simulink model "threephasePWMRectifier_open"  (R2017b)
settings: Solver=ode23  StartTime=0.0  StopTime=0.3  RelTol=1e-3  EnableMultiTasking=on
undefined symbols (not defined in the file): DiscIntNeverNeededParam, Vdc_Ref
libraries: powerlib x15, powerlib_extras x7, simulink x2
settings Model: Creator=ztm  LastModifiedBy=陈鹏旺
settings DataIOCC: LimitDataPoints=on  SaveFormat=Array  SignalLoggingSaveFormat=ModelDataLogs
settings OptimizationCC: ExpressionDepthLimit=2147483647  LifeSpan=inf
settings DebuggingCC: UnderspecifiedInitializationDetection=Classic  MergeDetectMultiDrivingBlocksExec=none  SolverPrmCheckMsg=warning  FcnCallInpInsideContextMsg=warning  StateNameClashWarn=warning  SFUnexpectedBacktrackingDiag=warning  SFNoUnconditionalDefaultTransitionDiag=warning  SFExecutionAtInitializationDiag=none
settings HardwareCC: ProdBitPerPointer=32  ProdBitPerSizeT=32  ProdBitPerPtrDiffT=32  ProdLargestAtomicFloat=None  ProdIntDivRoundTo=Undefined  ProdEndianess=Unspecified  ProdWordSize=32  ProdHWDeviceType=32-bit Generic
settings ModelReferenceCC: PropagateSignalLabelsOutOfModel=off
settings CodeAppCC: StateflowObjectComments=on
settings GRTTargetCC: TargetLangStandard=C89/C90 (ANSI)  GeneratePreprocessorConditionals=Disable all  CombineOutputUpdateFcns=off  GRTInterface=on
settings ConfigComp: CovMetricSettings=dw  CovHtmlReporting=on  CovSaveCumulativeToWorkspaceVar=on  CovSaveSingleToWorkspaceVar=on  CovExternalEMLEnable=off
settings SimscapeCC: SimscapeNormalizeSystem=off

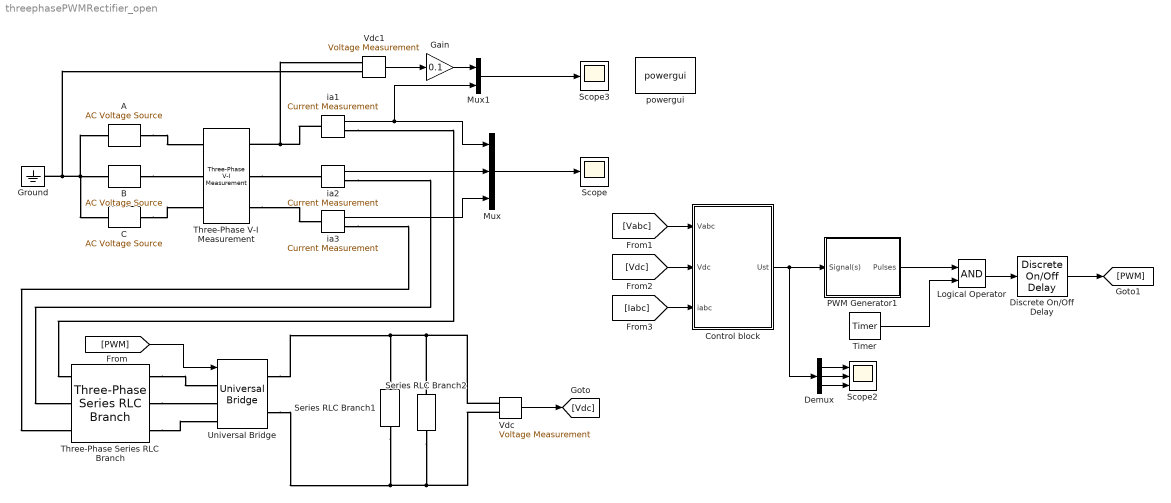
== system threephasePWMRectifier_open ==
  A : powerlib/Electrical Sources/AC Voltage Source  Amplitude=130*sqrt(2)/sqrt(3)  Phase=0  Frequency=50  SampleTime=0  Measurements=Voltage  BusType=swing  Pref=10e3  Qref=0  Qmin=-inf  Qmax=+inf
  B : powerlib/Electrical Sources/AC Voltage Source  Amplitude=130*sqrt(2)/sqrt(3)  Phase=-120  Frequency=50  SampleTime=0  Measurements=Voltage  BusType=swing  Pref=10e3  Qref=0  Qmin=-inf  Qmax=+inf
  C : powerlib/Electrical Sources/AC Voltage Source  Amplitude=130*sqrt(2)/sqrt(3)  Phase=120  Frequency=50  SampleTime=0  Measurements=Voltage  BusType=swing  Pref=10e3  Qref=0  Qmin=-inf  Qmax=+inf
  Control block : Subsystem  mask(DC Regulator){Vdc_Ref=280, =Vdc_Ref, Par_VdcReg=[0.8 0.008], Par_IReg=[20 0.0001 0], Par_Nom=[130 605], Ts=1/9000/2, h_I=[10.5 0]}
      mask prompts: Vdc_Ref "DC Voltage setpoint (Volts)";  "DC Voltage setpoint (Volts)"; Par_VdcReg "Vdc Regulator Gains: [ Kp  Ki]"; Par_IReg "Current Regulators Gain: [ Kp Ki Kr ]"; Par_Nom "Nominal Voltage and power: [ Vnom (volts rms L-L)  Pnom (VA) ]"; Ts "Time Step (s)"; h_I "[kph kih]"
      mask init:
      | Vnom=Par_Nom(1);
      | Pnom=Par_Nom(2);
      | Kp_I=Par_IReg(1);
      | Ki_I=Par_IReg(2);
      | Kr=Par_IReg(3);
      | Kp_Vdc=Par_VdcReg(1);
      | Ki_Vdc=Par_VdcReg(2);
      | Kph_I=h_I(1);
      | Kih_I=h_I(2);
  Demux : Demux  Outputs=3
  Discrete On/Off Delay : powerlib_extras/Discrete  Control Blocks/Discrete On//Off Delay  type_delay=On delay  delay=5e-6  ic=0  Ts=3.9e-7
  Gain : Gain  Gain=0.1
  Ground : powerlib/Elements/Ground  LConnTagsString=a
  Logical Operator : Logic  AllPortsSameDT=off  OutDataTypeStr=boolean
  Mux : Mux  Inputs=3
  Mux1 : Mux  Inputs=2
  PWM Generator1 : Subsystem  AncestorBlock="powerlib_extras/Control  Blocks/PWM Generator"  DialogController=POWERSYS.PowerSysDialog  mask(PWM Generator){GeneratorMode=3-arm  bridge (6 pulses), Fc=9000, Internal=off, mIndex=0.2, Freq=50, Phase=60}
      mask prompts: GeneratorMode "Generator Mode"; Fc "Carrier frequency (Hz):"; Internal "Internal generation of modulating signal(s)"; mIndex "Modulation index  (0<m<1) :"; Freq "Frequency of output voltage (Hz)"; Phase "Phase of output voltage (degrees)"
      mask help:
      | This block generates pulses for carrier-based PWM (Pulse Width Modulation), self-commutated IGBTs,GTOs or FETs bridges.
      |
      | Depending on the number of bridge arms selected in the "Generator Mode" parameter, the block can be used either for single-phase or three-phase PWM control.
      mask init:
      | powericon('psbcallbacks',gcb,'PWM Generator');
      | if Freq==0
      |     Phase=90;
      | end
      | switch GeneratorMode
      | case 1,
      |     Internal_Phase=0;
      |    Signal_PortWidth=1;
      |    Select1_Elements=[1 2];
      |    Select1_PortWidth=2;
      |    Select3_Elements=[1 2];
      |    Select3_PortWidth=4;
      | case 2,
      |     Internal_Phase=0;
      |     Signal_PortWidth=1;
      |     Select1_Elements=[1 2];
      |     Select1_PortWidth=2;
      |     Select3_Elements=[1 2 3 4];
      |     Select3_PortWidth=4;
      | case 3,
      |     Internal_Phase=[0 -2*pi/3 2*pi/3];
      |     Signal_PortWidth=3;
      |     Select1_Elements=[1 4 2 5 3 6];
      |     Select1_PortWidth=6;
      |    Select3_Elements=[1 2 3 4 5 6];
      |    Select3_PortWidth=12;
      | case 4,
      |     Internal_Phase=[0 -2*pi/3 2*pi/3];
      |     Signal_PortWidth=3;
      |     Select1_Elements=[1 4 2 5 3 6];
      |     Select1_PortWidth=6;
      |    Select3_Elements=[1 2 3 4 5 6 7 8 9 10 11 12];
      |    Select3_PortWidth=12;
      | end
      | power_initmask();
      mask Help: web(psbhelp)
      mask TypeOptions GeneratorMode: 1-arm  bridge (2 pulses) | 2-arm  bridge (4 pulses) | 3-arm  bridge (6 pulses) | Double 3-arm  bridges (12 pulses)
  Scope : Scope
  Scope2 : Scope  NumInputPorts=3
  Scope3 : Scope
  Series RLC Branch1 : powerlib/Elements/Series RLC Branch  LConnTagsString=__new0  RConnTagsString=__new0  BranchType=C  Resistance=20  Inductance=1e-5  SetiL0=off  InitialCurrent=0  Capacitance=2e-3  Setx0=on  InitialVoltage=252  Measurements=None
  Series RLC Branch2 : powerlib/Elements/Series RLC Branch  LConnTagsString=__new0  RConnTagsString=__new0  BranchType=R  Resistance=60  Inductance=1e-5  SetiL0=off  InitialCurrent=0  Capacitance=1e-6  Setx0=off  InitialVoltage=0  Measurements=None
  Three-Phase Series RLC Branch : powerlib/Elements/Three-Phase Series RLC Branch  LConnTagsString=A|B|C  RConnTagsString=A|B|C  BranchType=RL  Resistance=1e-4  Inductance=2e-3  Capacitance=1e-6  Measurements=None
  Three-Phase V-I Measurement : powerlib/Measurements/Three-Phase V-I Measurement  VoltageMeasurement=phase-to-ground  SetLabelV=on  LabelV=Vabc  Vpu=off  VpuLL=off  CurrentMeasurement=yes  SetLabelI=on  LabelI=Iabc  Ipu=off  Pbase=100e6  Vbase=500e3  OutputType=Complex  PhasorSimulation=off  PSBequivalent=0
  Timer : powerlib_extras/Control  Blocks/Timer  t=[0 0.001]  e=[0 1]
  Universal Bridge : powerlib/Power Electronics/Universal Bridge  Arms=3  SnubberResistance=1e6  SnubberCapacitance=inf  Device=MOSFET / Diodes  Ron=11e-3  Lon=0  ForwardVoltages="[  0  0  ]"  ForwardVoltage=0  GTOparameters=[ 10e-6 , 20e-6 ]  IGBTparameters=[ 1e-6 , 2e-6 ]  Measurements=None  Measurements_2=None  converterType=Rectifier
  Vdc : powerlib/Measurements/Voltage Measurement  PhasorSimulation=off  OutputType=Complex  PSBequivalent=0
  Vdc1 : powerlib/Measurements/Voltage Measurement  PhasorSimulation=off  OutputType=Complex  PSBequivalent=0
  ia1 : powerlib/Measurements/Current Measurement  PhasorSimulation=off  OutputType=Complex  PSBequivalent=0
  ia2 : powerlib/Measurements/Current Measurement  PhasorSimulation=off  OutputType=Complex  PSBequivalent=0
  ia3 : powerlib/Measurements/Current Measurement  PhasorSimulation=off  OutputType=Complex  PSBequivalent=0
  powergui : powerlib/powergui  Priority=1  SimulationMode=Discrete  SampleTime=3.9e-7  frequency=60  Iterations=50  frequencyindice=50  Pbase=100e6  ErrMax=1e-4  UnitsV=kV  UnitsW=MW  buscounter=0  FunctionMessages=off  echomessages=off  EnableUseOfTLC=off  CurrentSourceSwitches=off  DisableSnubberDevices=off  DisableRonSwitches=off  DisableVfSwitches=off  DisplayEquations=off  SolverType=Tustin/Backward Euler (TBE)  Interpol=off  ExternalGateDelay=off  methode=off  Ts=0  x0status=blocks  SPID=off  SwTol=0  HookPort=off  RestoreLinks=warning  ResistiveCurrentMeasurement=off  Frange=[0:2:500]  Ylog=off  Xlog=on  ShowGrid=off  save=off  variable=ZData  structure=ScopeData  ZoomFFT=off  StartTime=0.15  cycles=3  DisplayStyle=2  fundamental=50  FreqAxis=off  MaxFrequency=9000  frequencyindicesteady=1  RmsSteady=1  display=off
  wires:
  Vdc/1 -> [Vdc]
  Mux/1 -> Scope/1
  [Vabc] -> Control block/1(Vabc)
  [Vdc] -> Control block/2(Vdc)
  [Iabc] -> Control block/3(iabc)
  Control block/1(Ust) -> Demux/1, PWM Generator1/1(Signal(s))
  Demux/1 -> Scope2/1
  Demux/2 -> Scope2/2
  Demux/3 -> Scope2/3
  Timer/1 -> Logical Operator/2
  Logical Operator/1 -> Discrete On/Off Delay/1
  Vdc1/1 -> Gain/1
  Gain/1 -> Mux1/1
  Mux1/1 -> Scope3/1
  ia1/1 -> Mux/1, Mux1/2
  ia3/1 -> Mux/3
  ia2/1 -> Mux/2
  Discrete On/Off Delay/1 -> [PWM]
  PWM Generator1/1(Pulses) -> Logical Operator/1
  [PWM] -> Universal Bridge/1
  connections:
  C/LConn1 -- B/LConn1 -- A/LConn1 -- Ground/LConn1 -- Vdc1/LConn2
  B/RConn1 -- Three-Phase V-I Measurement/LConn2
  A/RConn1 -- Three-Phase V-I Measurement/LConn1
  C/RConn1 -- Three-Phase V-I Measurement/LConn3
  ia1/LConn1 -- Three-Phase V-I Measurement/RConn1 -- Vdc1/LConn1
  Three-Phase V-I Measurement/RConn3 -- ia3/LConn1
  Three-Phase V-I Measurement/RConn2 -- ia2/LConn1
  Vdc/LConn2 -- Series RLC Branch2/RConn1 -- Universal Bridge/RConn2 -- Series RLC Branch1/RConn1
  Three-Phase Series RLC Branch/RConn1 -- Universal Bridge/LConn1
  Three-Phase Series RLC Branch/RConn2 -- Universal Bridge/LConn2
  Three-Phase Series RLC Branch/RConn3 -- Universal Bridge/LConn3
  ia1/RConn1 -- Three-Phase Series RLC Branch/LConn1
  ia2/RConn1 -- Three-Phase Series RLC Branch/LConn2
  ia3/RConn1 -- Three-Phase Series RLC Branch/LConn3
  Vdc/LConn1 -- Series RLC Branch2/LConn1 -- Series RLC Branch1/LConn1 -- Universal Bridge/RConn1

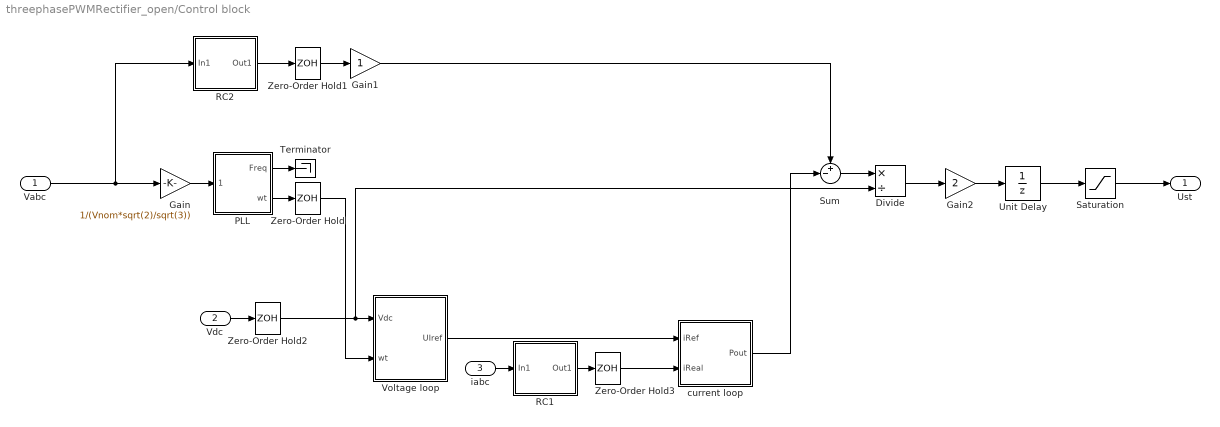
== system threephasePWMRectifier_open/Control block ==
  Vabc : Inport
  Vdc : Inport  Port=2
  iabc : Inport  Port=3
  Divide : Product  Inputs=*/
  Gain : Gain  Gain=1/(Vnom*sqrt(2)/sqrt(3))
  Gain1 : Gain
  Gain2 : Gain  Gain=2
  PLL : Subsystem  AncestorBlock=|  mask(Discrete 3-phase PLL){Fmin=-48, Par_Init=[0 50], ParK=[100 140], Ts=Ts, AGC=off}
      | powerlib_extras/Discrete 
      | Control Blocks/Discrete
      | 3-phase PLL
      mask prompts: Fmin "Minimum frequency (Hz):"; Par_Init "Initial inputs:[ Phase(degrees)   Frequency(Hz) ]"; ParK "Regulator gains [ Kp  Ki  Kd ]"; Ts "Sample time:"; AGC "Enable Automatic Gain Control"
      mask help:
      | This Phase Locked Loop (PLL) system can be used  to synchronize on a set of variable frequency, three-phase sinusoidal signals. If the Automatic Gain Control is enabled, the input (phase error) of the PLL regulator is scaled according to the input signals magnitude.
      |
      | For optimal performance, the following settings are recommended:
      |   [ Kp Ki  Kd ] = [ 180  3200  1 ]
      |   "Enable Automatic Gain Control" checked
      |
      | Input 1: Vector containing the normalized three-phase signals [Va Vb Vc]
      | Output 1:  Measured frequency (Hz) = w/(2pi)
      | Output 2:  Ramp w.t varying between  0 and 2*pi,
      |      synchronized on zero crossings of the fundamental (positive-sequence) of phase A.
      | Output 3: Vector [sin(wt) cos(wt)]
      mask init:
      | Kp=ParK(1);
      | Ki=ParK(2);
      | if length(ParK)==2
      |     Kd=0;
      | else
      |     Kd=ParK(3);
      | end    
      | Phase_Init=Par_Init(1);
      | Finit=Par_Init(2);
      | power_initmask();
      settings: OpenFcn=power_openblockproxy();
  RC1 : Subsystem
  RC2 : Subsystem
  Saturation : Saturate  UpperLimit=0.98  LowerLimit=-0.98
  Sum : Sum  Inputs=+-|
  Terminator : Terminator
  Unit Delay : UnitDelay  SampleTime=Ts/2
  Voltage loop : Subsystem
  Zero-Order Hold{,1..3} (4 alike) : ZeroOrderHold  SampleTime=Ts
  current loop : Subsystem
  Ust : Outport
  wires:
  Gain/1 -> PLL/1(Vabc(pu))
  PLL/1(Freq) -> Terminator/1
  PLL/2(wt) -> Zero-Order Hold/1
  RC2/1(Out1) -> Zero-Order Hold1/1
  Zero-Order Hold1/1 -> Gain1/1
  Vdc/1 -> Zero-Order Hold2/1
  Zero-Order Hold/1 -> Voltage loop/2(wt)
  Zero-Order Hold2/1 -> Voltage loop/1(Vdc), Divide/2
  iabc/1 -> RC1/1(In1)
  RC1/1(Out1) -> Zero-Order Hold3/1
  Gain1/1 -> Sum/1
  Sum/1 -> Divide/1
  Divide/1 -> Gain2/1
  Gain2/1 -> Unit Delay/1
  Saturation/1 -> Ust/1
  Vabc/1 -> Gain/1, RC2/1(In1)
  Zero-Order Hold3/1 -> current loop/2(iReal)
  Unit Delay/1 -> Saturation/1
  current loop/1(Pout) -> Sum/2
  Voltage loop/1(UIref) -> current loop/1(iRef)

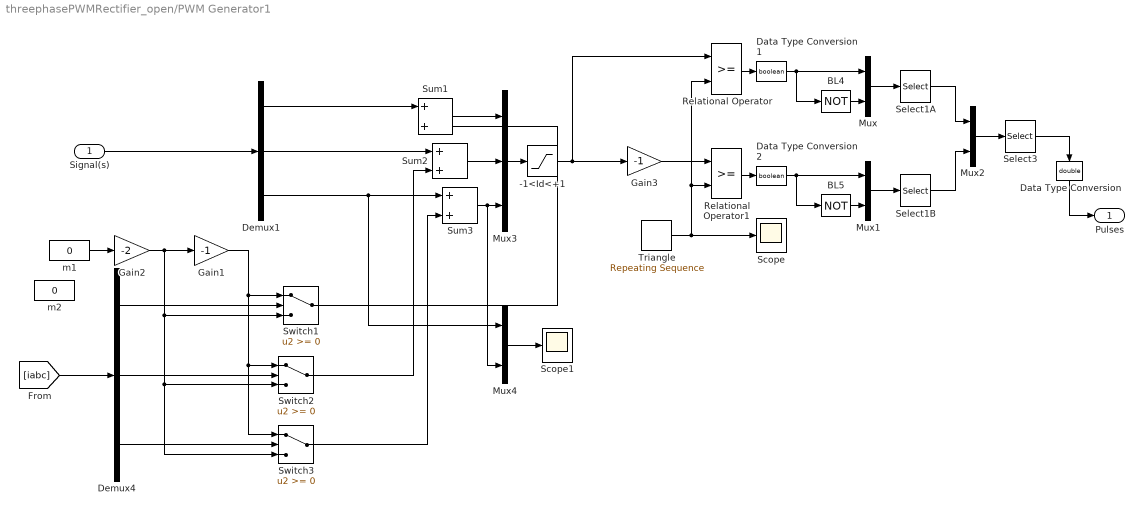
== system threephasePWMRectifier_open/PWM Generator1 ==
  Signal(s) : Inport
  -1<Id<+1 : Saturate  UpperLimit=0.94  LowerLimit=-0.94
  BL4 : Logic  Operator=NOT  Inputs=1
  BL5 : Logic  Operator=NOT  Inputs=1
  Data Type Conversion : DataTypeConversion  OutDataTypeStr=double  SaturateOnIntegerOverflow=on  RndMeth=Zero
  Data Type Conversion1 : DataTypeConversion  OutDataTypeStr=boolean  SaturateOnIntegerOverflow=on  RndMeth=Zero
  Data Type Conversion2 : DataTypeConversion  OutDataTypeStr=boolean  SaturateOnIntegerOverflow=on  RndMeth=Zero
  Demux1 : Demux  Outputs=3
  Demux4 : Demux  Outputs=3
  Gain1 : Gain  Gain=-1  SaturateOnIntegerOverflow=on  OutDataTypeStr=Inherit: Same as input  ParamDataTypeStr=Inherit: Same as input
  Gain2 : Gain  Gain=-2  SaturateOnIntegerOverflow=on  OutDataTypeStr=Inherit: Same as input  ParamDataTypeStr=Inherit: Same as input
  Gain3 : Gain  Gain=-1  SaturateOnIntegerOverflow=on  OutDataTypeStr=Inherit: Same as input  ParamDataTypeStr=Inherit: Same as input
  Mux{,1..2,4} (4 alike) : Mux  Inputs=2
  Mux3 : Mux  Inputs=3
  Relational Operator : RelationalOperator  RndMeth=Nearest  InputSameDT=on
  Relational Operator1 : RelationalOperator  RndMeth=Nearest  InputSameDT=on
  Scope : Scope
  Scope1 : Scope
  Select1A : Selector  InputPortWidth=Select1_PortWidth  IndexOptions=Index vector (dialog)  Indices=Select1_Elements  OutputSizes=1
  Select1B : Selector  InputPortWidth=Select1_PortWidth  IndexOptions=Index vector (dialog)  Indices=Select1_Elements  OutputSizes=1
  Select3 : Selector  InputPortWidth=Select3_PortWidth  IndexOptions=Index vector (dialog)  Indices=Select3_Elements  OutputSizes=1
  Sum1 : Sum  SaturateOnIntegerOverflow=on  InputSameDT=on  OutDataTypeStr=Inherit: Same as first input
  Sum2 : Sum  SaturateOnIntegerOverflow=on  InputSameDT=on  OutDataTypeStr=Inherit: Same as first input
  Sum3 : Sum  SaturateOnIntegerOverflow=on  InputSameDT=on  OutDataTypeStr=Inherit: Same as first input
  Switch1 : Switch  InputSameDT=on
  Switch2 : Switch  InputSameDT=on
  Switch3 : Switch  InputSameDT=on
  Triangle : simulink/Sources/Repeating Sequence  rep_seq_t=[0 1/Fc/4 3/Fc/4 1/Fc]  rep_seq_y=[0 -1 1 0]
  m1 : Constant  Value=0
  m2 : Constant  Value=0
  Pulses : Outport
  wires:
  Data Type Conversion2/1 -> Mux1/1, BL5/1
  Relational Operator1/1 -> Data Type Conversion2/1
  Data Type Conversion1/1 -> Mux/1, BL4/1
  Relational Operator/1 -> Data Type Conversion1/1
  Data Type Conversion/1 -> Pulses/1
  Select3/1 -> Data Type Conversion/1
  Gain3/1 -> Relational Operator1/1
  BL4/1 -> Mux/2
  BL5/1 -> Mux1/2
  Mux/1 -> Select1A/1
  Mux1/1 -> Select1B/1
  Select1A/1 -> Mux2/1
  Select1B/1 -> Mux2/2
  Mux2/1 -> Select3/1
  Triangle/1 -> Relational Operator1/2, Relational Operator/2, Scope/1
  [iabc] -> Demux4/1
  Demux4/1 -> Switch1/2
  Gain1/1 -> Switch1/1, Switch2/1, Switch3/1
  Demux4/2 -> Switch2/2
  Demux4/3 -> Switch3/2
  Signal(s)/1 -> Demux1/1
  Mux3/1 -> -1<Id<+1/1
  Switch1/1 -> Sum1/2
  Demux1/1 -> Sum1/1
  Sum1/1 -> Mux3/1
  Demux1/2 -> Sum2/1
  Demux1/3 -> Sum3/1, Mux4/1
  Sum3/1 -> Mux3/3, Mux4/2
  Sum2/1 -> Mux3/2
  Switch2/1 -> Sum2/2
  Switch3/1 -> Sum3/2
  -1<Id<+1/1 -> Gain3/1, Relational Operator/1
  Gain2/1 -> Gain1/1, Switch1/3, Switch3/3, Switch2/3
  Mux4/1 -> Scope1/1
  m1/1 -> Gain2/1

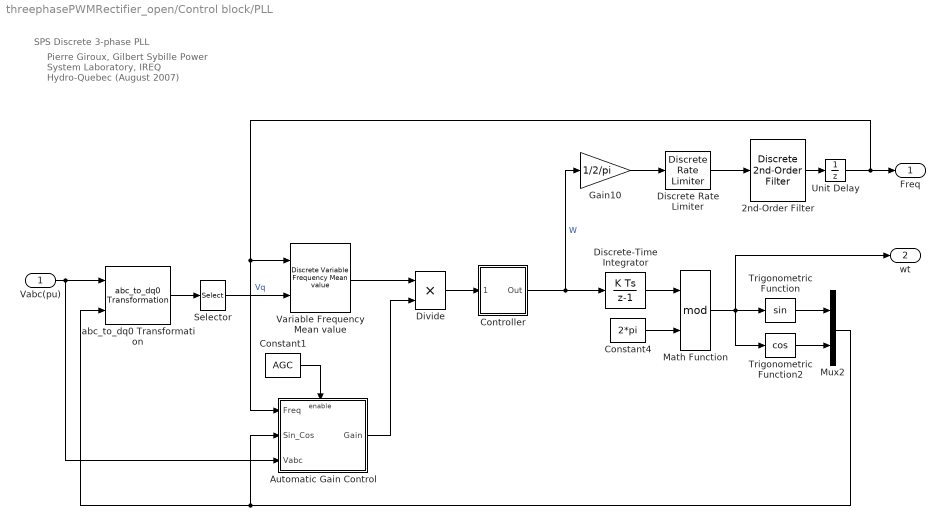
== system threephasePWMRectifier_open/Control block/PLL ==
  note: Pierre Giroux, Gilbert Sybille
      | Power System Laboratory, IREQ
      | Hydro-Quebec
      | (August 2007)
  note: SPS Discrete 3-phase PLL
  Vabc(pu) : Inport  PortDimensions=3
  2nd-Order Filter : powerlib_extras/Discrete  Control Blocks/Discrete  2nd-Order Filter  FilterType=Lowpass  Fo=25  Zeta=0.707  Ts=Ts  Initialize=on  Vac_Init=[0 0 Finit]  Vdc_Init=Finit  PlotResponse=off  param1=[1 500 0.1]
  Automatic Gain Control : Subsystem  TreatAsAtomicUnit=on
  Constant1 : Constant  Value=AGC
  Constant4 : Constant  Value=2*pi
  Controller : Subsystem  mask(Discrete PID Controller){Kp=Kp, Ki=Ki, Kd=Kd, Par_Limits=[10000 0], Init=2*pi*Finit, Ts=Ts}
      mask prompts: Kp "Proportional gain (Kp):"; Ki "Integral gain (Ki):"; Kd "Derivative gain (Kd):"; Par_Limits "Output limits: [ Upper   Lower ]"; Init "Output initial value:"; Ts "Sample time:"
      mask help: This block implements a discrete PID controller.
      mask init:
      | UpperLimit=Par_Limits(1);
      | LowerLimit=Par_Limits(2);
      | power_initmask();
      settings: OpenFcn=power_openblockproxy();
      mask Display: disp('PID');
  Discrete Rate Limiter : powerlib_extras/Discrete  Control Blocks/Discrete Rate Limiter  R=12  F=-12  Vinit=Finit  Ts=Ts
  Discrete-Time Integrator : DiscreteIntegrator  InitialCondition=Phase_Init*pi/180  SampleTime=Ts  ICPrevOutput=DiscIntNeverNeededParam  ICPrevScaledInput=DiscIntNeverNeededParam
  Divide : Product
  Gain10 : Gain  Gain=1/2/pi  SaturateOnIntegerOverflow=on  OutDataTypeStr=Inherit: Same as input  ParamDataTypeStr=Inherit: Same as input
  Math Function : Math  Operator=mod  SaturateOnIntegerOverflow=on
  Mux2 : Mux  Inputs=2
  Selector : Selector  InputPortWidth=3  IndexOptions=Index vector (dialog)  Indices=2  OutputSizes=1
  Trigonometric Function : Trigonometry
  Trigonometric Function2 : Trigonometry  Operator=cos
  Unit Delay : UnitDelay  InitialCondition=Finit  SampleTime=Ts
  Variable Frequency Mean value : powerlib_extras/Discrete Measurements/Discrete Variable Frequency Mean value  Finit=Finit  Fmin=Fmin  Vinit=0  Ts=Ts
  abc_to_dq0 Transformation : powerlib_extras/Measurements/abc_to_dq0 Transformation
  Freq : Outport
  wt : Outport  Port=2
  wires:
  Selector/1 -> Variable Frequency Mean value/2  "Vq"
  2nd-Order Filter/1 -> Unit Delay/1
  Unit Delay/1 -> Freq/1, Variable Frequency Mean value/1, Automatic Gain Control/1(Freq)
  Discrete Rate Limiter/1 -> 2nd-Order Filter/1
  Gain10/1 -> Discrete Rate Limiter/1
  Mux2/1 -> abc_to_dq0 Transformation/2, Automatic Gain Control/2(Sin_Cos)
  Trigonometric Function2/1 -> Mux2/2
  Trigonometric Function/1 -> Mux2/1
  Math Function/1 -> Trigonometric Function/1, wt/1, Trigonometric Function2/1
  Discrete-Time Integrator/1 -> Math Function/1
  Constant4/1 -> Math Function/2
  abc_to_dq0 Transformation/1 -> Selector/1
  Vabc(pu)/1 -> abc_to_dq0 Transformation/1, Automatic Gain Control/3(Vabc)
  Controller/1(Out) -> Discrete-Time Integrator/1, Gain10/1  "W"
  Variable Frequency Mean value/1 -> Divide/1
  Automatic Gain Control/1(Gain) -> Divide/2
  Divide/1 -> Controller/1(Error)
  Constant1/1 -> Automatic Gain Control/Enable

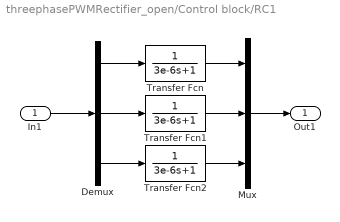
== system threephasePWMRectifier_open/Control block/RC1 ==
  In1 : Inport
  Demux : Demux  Outputs=3
  Mux : Mux  Inputs=3
  Transfer Fcn : TransferFcn  Denominator=[3e-6 1]
  Transfer Fcn1 : TransferFcn  Denominator=[3e-6 1]
  Transfer Fcn2 : TransferFcn  Denominator=[3e-6 1]
  Out1 : Outport
  wires:
  Mux/1 -> Out1/1
  Demux/3 -> Transfer Fcn2/1
  Transfer Fcn2/1 -> Mux/3
  Transfer Fcn1/1 -> Mux/2
  Demux/2 -> Transfer Fcn1/1
  Transfer Fcn/1 -> Mux/1
  Demux/1 -> Transfer Fcn/1
  In1/1 -> Demux/1

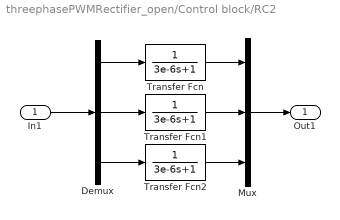
== system threephasePWMRectifier_open/Control block/RC2 ==
  In1 : Inport
  Demux : Demux  Outputs=3
  Mux : Mux  Inputs=3
  Transfer Fcn : TransferFcn  Denominator=[3e-6 1]
  Transfer Fcn1 : TransferFcn  Denominator=[3e-6 1]
  Transfer Fcn2 : TransferFcn  Denominator=[3e-6 1]
  Out1 : Outport
  wires:
  In1/1 -> Demux/1
  Demux/1 -> Transfer Fcn/1
  Transfer Fcn/1 -> Mux/1
  Demux/2 -> Transfer Fcn1/1
  Transfer Fcn1/1 -> Mux/2
  Transfer Fcn2/1 -> Mux/3
  Demux/3 -> Transfer Fcn2/1
  Mux/1 -> Out1/1

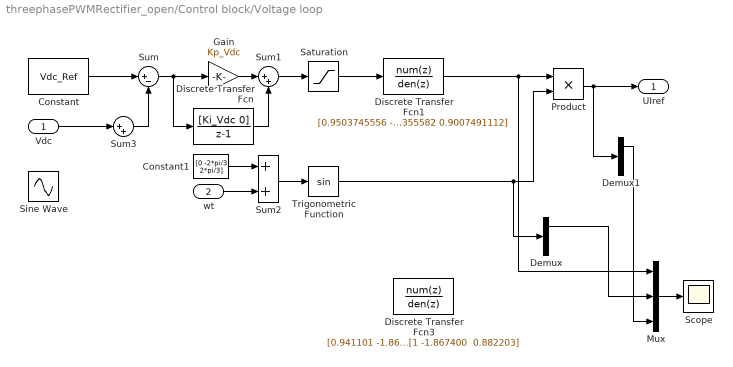
== system threephasePWMRectifier_open/Control block/Voltage loop ==
  Vdc : Inport
  wt : Inport  Port=2
  Constant : Constant  Value=Vdc_Ref
  Constant1 : Constant  Value=[0 -2*pi/3 2*pi/3]
  Demux : Demux  Outputs=3
  Demux1 : Demux  Outputs=3
  Discrete Transfer Fcn : DiscreteTransferFcn  Numerator=[Ki_Vdc 0]  Denominator=[1 -1]  SampleTime=Ts
  Discrete Transfer Fcn1 : DiscreteTransferFcn  Numerator=[0.9503745556 -1.890355582 0.9503745556]  Denominator=[1 -1.890355582 0.9007491112]  SampleTime=1/9000/2
  Discrete Transfer Fcn3 : DiscreteTransferFcn  Numerator=[0.941101 -1.867400 0.941101]  Denominator="[1 -1.867400  0.882203]"  SampleTime=1/9000/2
  Gain : Gain  Gain=Kp_Vdc  SampleTime=Ts
  Mux : Mux  Inputs=3
  Product : Product  SampleTime=4e-7  RndMeth=Zero
  Saturation : Saturate  UpperLimit=100  LowerLimit=-100
  Scope : Scope
  Sine Wave : Sin  Frequency=2*pi*50*3  SampleTime=0
  Sum : Sum  Inputs=|+-
  Sum1 : Sum  Inputs=|++
  Sum2 : Sum
  Sum3 : Sum  Inputs=|++
  Trigonometric Function : Trigonometry
  UIref : Outport
  wires:
  Constant/1 -> Sum/1
  Sum/1 -> Gain/1, Discrete Transfer Fcn/1
  Discrete Transfer Fcn/1 -> Sum1/2
  Gain/1 -> Sum1/1
  Sum1/1 -> Saturation/1
  Constant1/1 -> Sum2/1
  wt/1 -> Sum2/2
  Sum2/1 -> Trigonometric Function/1
  Trigonometric Function/1 -> Product/2, Demux/1
  Product/1 -> UIref/1, Demux1/1
  Demux1/1 -> Mux/3
  Demux/1 -> Mux/2
  Mux/1 -> Scope/1
  Saturation/1 -> Discrete Transfer Fcn1/1
  Vdc/1 -> Sum3/1
  Sum3/1 -> Sum/2
  Discrete Transfer Fcn1/1 -> Product/1, Mux/1

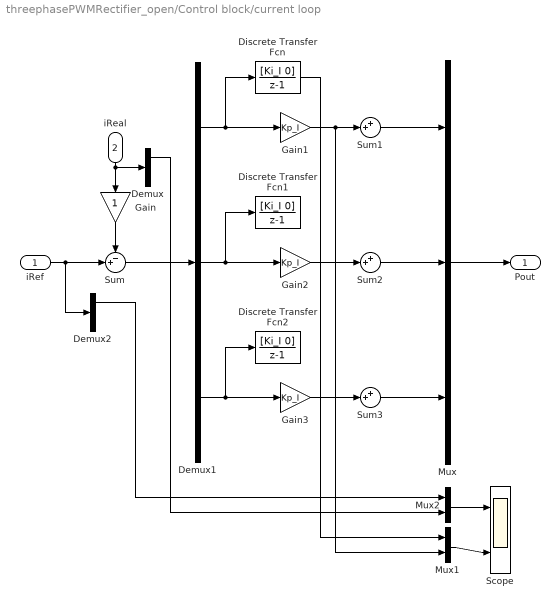
== system threephasePWMRectifier_open/Control block/current loop ==
  iRef : Inport
  iReal : Inport  Port=2
  Demux : Demux  Outputs=2
  Demux1 : Demux  Outputs=3
  Demux2 : Demux  Outputs=2
  Discrete Transfer Fcn : DiscreteTransferFcn  Numerator=[Ki_I 0]  Denominator=[1 -1]  SampleTime=Ts
  Discrete Transfer Fcn1 : DiscreteTransferFcn  Numerator=[Ki_I 0]  Denominator=[1 -1]  SampleTime=Ts
  Discrete Transfer Fcn2 : DiscreteTransferFcn  Numerator=[Ki_I 0]  Denominator=[1 -1]  SampleTime=Ts
  Gain : Gain
  Gain1 : Gain  Gain=Kp_I  SampleTime=Ts
  Gain2 : Gain  Gain=Kp_I  SampleTime=Ts
  Gain3 : Gain  Gain=Kp_I  SampleTime=Ts
  Mux : Mux  Inputs=3
  Mux1 : Mux  Inputs=2
  Mux2 : Mux  Inputs=2
  Scope : Scope  NumInputPorts=2
  Sum : Sum  Inputs=-+|  SampleTime=Ts
  Sum1 : Sum  Inputs=++|
  Sum2 : Sum  Inputs=++|
  Sum3 : Sum  Inputs=++|
  Pout : Outport
  wires:
  iReal/1 -> Gain/1, Demux/1
  Gain/1 -> Sum/1
  iRef/1 -> Sum/2, Demux2/1
  Sum/1 -> Demux1/1
  Demux1/1 -> Gain1/1, Discrete Transfer Fcn/1
  Discrete Transfer Fcn/1 -> Mux1/1
  Gain1/1 -> Sum1/2, Mux1/2
  Sum1/1 -> Mux/1
  Demux1/2 -> Discrete Transfer Fcn1/1, Gain2/1
  Gain2/1 -> Sum2/2
  Sum2/1 -> Mux/2
  Demux1/3 -> Gain3/1, Discrete Transfer Fcn2/1
  Gain3/1 -> Sum3/2
  Sum3/1 -> Mux/3
  Mux/1 -> Pout/1
  Demux2/1 -> Mux2/1
  Demux/1 -> Mux2/2
  Mux2/1 -> Scope/1
  Mux1/1 -> Scope/2

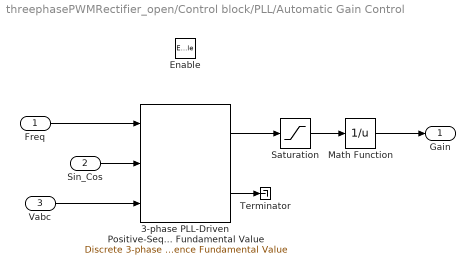
== system threephasePWMRectifier_open/Control block/PLL/Automatic Gain Control ==
  Freq : Inport
  Sin_Cos : Inport  Port=2
  Vabc : Inport  Port=3
  Enable : EnablePort  PropagateVarSize=During execution
  3-phase PLL-Driven Positive-Sequence Fundamental Value : powerlib_extras/Discrete Measurements/Discrete 3-phase PLL-Driven Positive-Sequence Fundamental Value  Finit=Finit  Fmin=Fmin  Par_Init=[1 0]  Ts=Ts
  Math Function : Math  Operator=reciprocal  SaturateOnIntegerOverflow=on
  Saturation : Saturate  UpperLimit=2  LowerLimit=0.01
  Terminator : Terminator
  Gain : Outport  InitialOutput=[1]
  wires:
  3-phase PLL-Driven Positive-Sequence Fundamental Value/2 -> Terminator/1
  Saturation/1 -> Math Function/1
  3-phase PLL-Driven Positive-Sequence Fundamental Value/1 -> Saturation/1
  Freq/1 -> 3-phase PLL-Driven Positive-Sequence Fundamental Value/1
  Sin_Cos/1 -> 3-phase PLL-Driven Positive-Sequence Fundamental Value/2
  Vabc/1 -> 3-phase PLL-Driven Positive-Sequence Fundamental Value/3
  Math Function/1 -> Gain/1

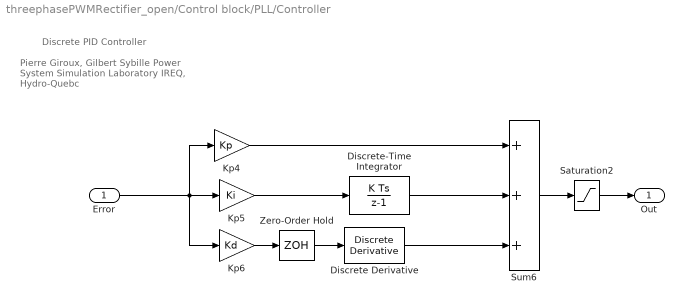
== system threephasePWMRectifier_open/Control block/PLL/Controller ==
  note: Pierre Giroux, Gilbert Sybille
      | Power System Simulation Laboratory
      | IREQ, Hydro-Quebc
  note: Discrete PID Controller
  Error : Inport
  Discrete Derivative : simulink/Discrete/Discrete Derivative  gainval=1.0  ICPrevScaledInput=0.0  InputProcessing=Inherited  OutMin=[]  OutMax=[]  OutDataType=sfix(16)  OutScaling=2^-10  DoSatur=off
  Discrete-Time Integrator : DiscreteIntegrator  InitialCondition=Init  SampleTime=Ts  LimitOutput=on  UpperSaturationLimit=UpperLimit  LowerSaturationLimit=LowerLimit  ICPrevOutput=DiscIntNeverNeededParam  ICPrevScaledInput=DiscIntNeverNeededParam
  Kp4 : Gain  Gain=Kp  SaturateOnIntegerOverflow=on  OutDataTypeStr=Inherit: Same as input  ParamDataTypeStr=Inherit: Same as input
  Kp5 : Gain  Gain=Ki  SaturateOnIntegerOverflow=on  OutDataTypeStr=Inherit: Same as input  ParamDataTypeStr=Inherit: Same as input
  Kp6 : Gain  Gain=Kd  SaturateOnIntegerOverflow=on  OutDataTypeStr=Inherit: Same as input  ParamDataTypeStr=Inherit: Same as input
  Saturation2 : Saturate  UpperLimit=UpperLimit  LowerLimit=LowerLimit
  Sum6 : Sum  Inputs=+++  SaturateOnIntegerOverflow=on  InputSameDT=on  OutDataTypeStr=Inherit: Same as first input
  Zero-Order Hold : ZeroOrderHold  SampleTime=Ts
  Out : Outport  InitialOutput=0
  wires:
  Error/1 -> Kp4/1, Kp5/1, Kp6/1
  Sum6/1 -> Saturation2/1
  Kp5/1 -> Discrete-Time Integrator/1
  Kp6/1 -> Zero-Order Hold/1
  Kp4/1 -> Sum6/1
  Discrete-Time Integrator/1 -> Sum6/2
  Discrete Derivative/1 -> Sum6/3
  Saturation2/1 -> Out/1
  Zero-Order Hold/1 -> Discrete Derivative/1
